simulink model "HeadlessPositionControllerVariableQuadDynamicsMdl"  (R2016b)
settings: Solver=FixedStepAuto  StartTime=0.0  StopTime=10  FixedStep=1/1000  RelTol=1e-3  EnableMultiTasking=on
undefined symbols (not defined in the file): Params, QuaternionController_nav
libraries: simulink x4
settings Model: Creator=Raj  LastModifiedBy=Hans
settings DataIOCC: LimitDataPoints=on  SaveFormat=Array
settings OptimizationCC: LifeSpan=inf
settings DebuggingCC: UnderspecifiedInitializationDetection=Classic  MergeDetectMultiDrivingBlocksExec=none  SolverPrmCheckMsg=warning  StateNameClashWarn=warning  SFUnexpectedBacktrackingDiag=warning  SFNoUnconditionalDefaultTransitionDiag=warning  SFExecutionAtInitializationDiag=none
settings HardwareCC: ProdBitPerPointer=32  ProdBitPerSizeT=32  ProdBitPerPtrDiffT=32  ProdLargestAtomicFloat=None  ProdIntDivRoundTo=Undefined  ProdEndianess=Unspecified  ProdWordSize=32  ProdHWDeviceType=32-bit Generic
settings ModelReferenceCC: PropagateSignalLabelsOutOfModel=off
settings GRTTargetCC: TargetLangStandard=C89/C90 (ANSI)  GeneratePreprocessorConditionals=Disable all
settings ConfigComp: CovMetricSettings=dw  CovHtmlReporting=on  CovSaveCumulativeToWorkspaceVar=on  CovSaveSingleToWorkspaceVar=on  CovExternalEMLEnable=off  CovSFcnEnable=off

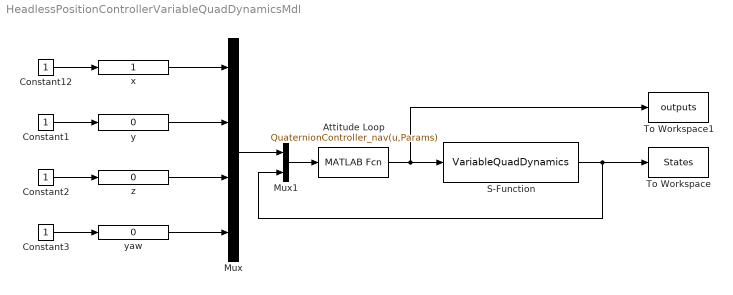
== system HeadlessPositionControllerVariableQuadDynamicsMdl ==
  Attitude Loop : MATLABFcn  MATLABFcn=QuaternionController_nav(u,Params)  OutputDimensions=4
  Constant{1..3,12} (4 alike) : Constant
  Mux : Mux
  Mux1 : Mux  Inputs=2
  S-Function : S-Function  FunctionName=VariableQuadDynamics  Parameters=Params  SFunctionDeploymentMode=off  EnableBusSupport=off
  To Workspace : ToWorkspace  VariableName=States  SaveFormat=Timeseries  SampleTime=-1
  To Workspace1 : ToWorkspace  VariableName=outputs  SaveFormat=Timeseries  SampleTime=-1
  x : simulink/Math Operations/Slider Gain  low=-20  gain=1  high=100
  y : simulink/Math Operations/Slider Gain  low=-10  gain=0  high=10
  yaw : simulink/Math Operations/Slider Gain  low=-10  gain=0  high=10
  z : simulink/Math Operations/Slider Gain  low=-10  gain=0  high=10
  wires:
  Constant12/1 -> x/1
  Constant1/1 -> y/1
  Constant2/1 -> z/1
  S-Function/1 -> Mux1/2, To Workspace/1
  z/1 -> Mux/3
  y/1 -> Mux/2
  x/1 -> Mux/1
  Attitude Loop/1 -> S-Function/1, To Workspace1/1
  Mux1/1 -> Attitude Loop/1
  Mux/1 -> Mux1/1
  Constant3/1 -> yaw/1
  yaw/1 -> Mux/4
